simulink model "third"  (Simulink 8.6)
settings: Solver=ode23tb  StartTime=0.0  StopTime=3  MaxStep=1e-5  RelTol=1e-3
libraries: powerlib x6, simulink x2, powerlib_extras x1
settings Model: Creator=lenovo  LastModifiedBy=Administrator
settings OptimizationCC: InitFltsAndDblsToZero=on
settings DebuggingCC: SaveWithParameterizedLinksMsg=none  SignalResolutionControl=TryResolveAllWithWarning  MultiTaskDSMMsg=warning  MultiTaskCondExecSysMsg=none  FcnCallInpInsideContextMsg=UseLocalSettings
settings GRTTargetCC: TargetFcnLib=ansi_tfl_tmw.mat

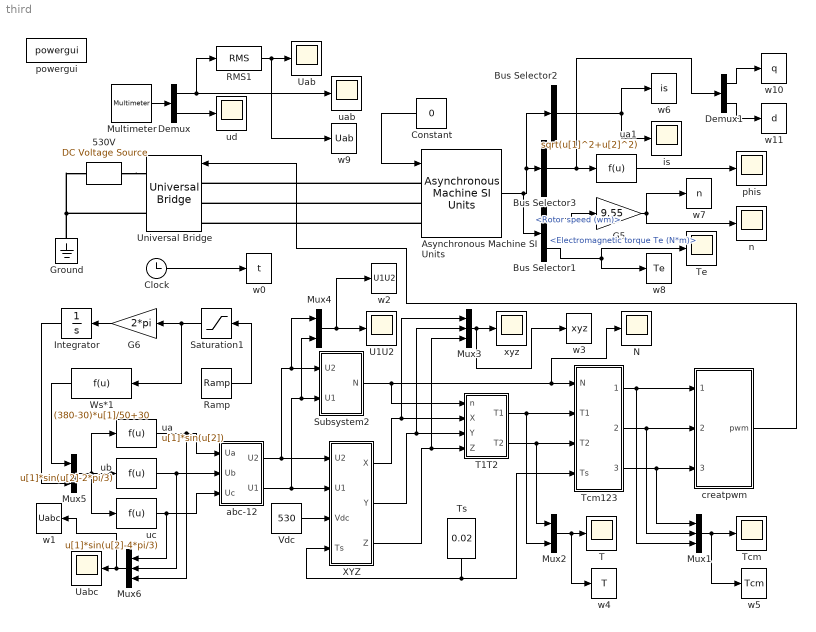
== system third ==
  530V : powerlib/Electrical Sources/DC Voltage Source  Amplitude=530  Measurements=Voltage
  Asynchronous Machine SI Units : powerlib/Machines/Asynchronous Machine SI Units  RotorType=Squirrel-cage  PresetModel=No  MechanicalLoad=Torque Tm  ShowDetailedParameters=on  ReferenceFrame=Rotor  Units=SI  MeasurementBus=off  NominalParameters=[2200 380 50]  Stator=[6.9 0.0455]  Rotor=[8.18 0.0455]  Cage1=[0.4155 0.002066]  Cage2=[0.4168 0.0003495]  Lm=1.0039  Mechanical=[0.02 0.005752 2]  PolePairs=2  InitialConditions="[ 1,0   0,0,0   0,0,0 ]"  SimulateSaturation=off  Saturation=[9.9249,19.6672,38.0377,51.3988,69.2824,105.1337,152.5532,214.2421,303.1917;230, 322, 414, 460, 506, 552, 598, 644, 690]  LoadFlowParameters=0  TsPowergui=0  TsBlock=-1  IterativeModel=Forward Euler  Pmec=1.492e+006
  Bus Selector1 : BusSelector  OutputSignals=Mechanical.Rotor speed (wm),Mechanical.Electromagnetic torque Te (N*m)
  Bus Selector2 : BusSelector  OutputSignals=Stator measurements.Stator current is_a (A),Stator measurements.Stator current is_b (A),Stator measurements.Stator current is_c (A)  OutputAsBus=on
  Bus Selector3 : BusSelector  OutputSignals=Stator measurements.Stator flux phis_q (V s),Stator measurements.Stator flux phis_d (V s)  OutputAsBus=on
  Clock : Clock
  Constant : Constant  Value=0
  Demux : Demux  Outputs=2
  Demux1 : Demux  Outputs=2
  G5 : Gain  Gain=9.55
  G6 : Gain  Gain=2*pi
  Ground : powerlib/Elements/Ground  LConnTagsString=a
  Integrator : Integrator
  Multimeter : powerlib/Measurements/Multimeter  PhasorSimulation=off  OutputType=Complex  sel=[7 11]  L=17  Gain=[1 1]  yselected={'Uab: Universal Bridge','Usrc: 530V'};  PSBOutputType=1  PSBequivalent=0  AxesSetting=[0,0.1,-100,100]  Display=0  SavedBlockNames=-11
  Mux1 : Mux  Inputs=3
  Mux2 : Mux  Inputs=2
  Mux3 : Mux  Inputs=3
  Mux4 : Mux  Inputs=2
  Mux5 : Mux  Inputs=2
  Mux6 : Mux  Inputs=3
  N : Scope
  RMS1 : powerlib_extras/Measurements/RMS  f1=60
  Ramp : simulink/Sources/Ramp  slope=50  start=0  X0=0
  Saturation1 : Saturate  UpperLimit=50
  Subsystem2 : Subsystem
  T : Scope
  T1T2 : Subsystem
  Tcm : Scope
  Tcm123 : Subsystem
  Te : Scope
  Ts : Constant  Value=0.02
  U1U2 : Scope
  Uab : Scope
  Uabc : Scope
  Universal Bridge : powerlib/Power Electronics/Universal Bridge  Arms=3  SnubberResistance=1e5  SnubberCapacitance=inf  Device=IGBT / Diodes  Ron=1e-3  Lon=0  ForwardVoltages="[  0  0  ]"  ForwardVoltage=0  GTOparameters=[ 10e-6 , 20e-6 ]  IGBTparameters=[ 1e-6 , 2e-6 ]  Measurements=All voltages and currents  Measurements_2=None  converterType=Rectifier
  Vdc : Constant  Value=530
  Ws*1 : Fcn  Expr=(380-30)*u[1]/50+30
  XYZ : Subsystem
  abc-12 : Subsystem
  creatpwm : Subsystem
  is : Scope
  n : Scope
  phis : Scope
  powergui : powerlib/powergui  SimulationMode=Continuous  SolverType=Tustin/Backward Euler (TBE)  SampleTime=1e-5  frequency=60  SPID=off  DisableSnubberDevices=off  DisableRonSwitches=off  DisableVfSwitches=off  SwTol=0  DisplayEquations=off  Interpol=off  ExternalGateDelay=off  methode=off  Ts=0  FunctionMessages=off  echomessages=off  HookPort=off  EnableUseOfTLC=off  x0status=blocks  frequencyindice=50  Pbase=100e6  ErrMax=1e-4  Iterations=50  UnitsV=kV  UnitsW=MW  buscounter=0  RestoreLinks=warning  ResistiveCurrentMeasurement=off  Frange=[0:2:500]  Ylog=off  Xlog=on  ShowGrid=off  save=off  variable=ZData  ZoomFFT=on  StartTime=0.0  cycles=1  DisplayStyle=1  fundamental=60  FreqAxis=off  MaxFrequency=1000  frequencyindicesteady=1  RmsSteady=1  display=off
  ua : Fcn  Expr=u[1]*sin(u[2])
  ua1 : Fcn  Expr=sqrt(u[1]^2+u[2]^2)
  uab : Scope
  ub : Fcn  Expr=u[1]*sin(u[2]-2*pi/3)
  uc : Fcn  Expr=u[1]*sin(u[2]-4*pi/3)
  ud : Scope
  w0 : ToWorkspace  VariableName=t  SampleTime=-1
  w1 : ToWorkspace  VariableName=Uabc  SampleTime=-1
  w10 : ToWorkspace  VariableName=q  SampleTime=-1
  w11 : ToWorkspace  VariableName=d  SampleTime=-1
  w2 : ToWorkspace  VariableName=U1U2  SampleTime=-1
  w3 : ToWorkspace  VariableName=xyz  SampleTime=-1
  w4 : ToWorkspace  VariableName=T  SampleTime=-1
  w5 : ToWorkspace  VariableName=Tcm  SampleTime=-1
  w6 : ToWorkspace  VariableName=is  SampleTime=-1
  w7 : ToWorkspace  VariableName=n  SampleTime=-1
  w8 : ToWorkspace  VariableName=Te  SampleTime=-1
  w9 : ToWorkspace  VariableName=Uab  SampleTime=-1
  xyz : Scope
  wires:
  Multimeter/1 -> Demux/1
  Demux/1 -> RMS1/1, uab/1
  Demux/2 -> ud/1
  Bus Selector2/1 -> is/1, w6/1
  Bus Selector1/1 -> G5/1  "<Rotor speed (wm)>"
  G5/1 -> w7/1, n/1
  Bus Selector1/2 -> Te/1, w8/1  "<Electromagnetic torque Te (N*m)>"
  Constant/1 -> Asynchronous Machine SI Units/1
  Ramp/1 -> Saturation1/1
  G6/1 -> Integrator/1
  Ws*1/1 -> Mux5/1
  Integrator/1 -> Mux5/2
  Mux5/1 -> ub/1, ua/1, uc/1
  Ts/1 -> XYZ/4(Ts), Tcm123/4(Ts)
  Vdc/1 -> XYZ/3(Vdc)
  Subsystem2/1(N) -> T1T2/1(n), Tcm123/1(N), N/1
  XYZ/1(X) -> T1T2/2(X), Mux3/1
  XYZ/2(Y) -> T1T2/3(Y), Mux3/2
  XYZ/3(Z) -> T1T2/4(Z), Mux3/3
  T1T2/1(T1) -> Tcm123/2(T1), Mux2/2
  T1T2/2(T2) -> Tcm123/3(T2), Mux2/1
  Tcm123/1(Tcm1) -> creatpwm/1(Tcm1), Mux1/3
  Tcm123/2(Tcm2) -> creatpwm/2(Tcm2), Mux1/2
  Tcm123/3(Tcm3) -> creatpwm/3(Tcm3), Mux1/1
  ua/1 -> abc-12/1(Ua), Mux6/3
  ub/1 -> abc-12/2(Ub), Mux6/2
  uc/1 -> abc-12/3(Uc), Mux6/1
  RMS1/1 -> Uab/1, w9/1
  abc-12/1(U2) -> XYZ/1(U2), Subsystem2/1(U2), Mux4/1
  abc-12/2(U1) -> XYZ/2(U1), Subsystem2/2(U1), Mux4/2
  Saturation1/1 -> G6/1, Ws*1/1
  Mux1/1 -> Tcm/1, w5/1
  Mux2/1 -> T/1, w4/1
  Mux3/1 -> w3/1, xyz/1
  Mux4/1 -> U1U2/1, w2/1
  Mux6/1 -> Uabc/1, w1/1
  Clock/1 -> w0/1
  ua1/1 -> phis/1
  creatpwm/1(pwm) -> Universal Bridge/1
  Bus Selector3/1 -> ua1/1, Demux1/1
  Demux1/1 -> w10/1
  Demux1/2 -> w11/1
  Asynchronous Machine SI Units/1 -> Bus Selector1/1, Bus Selector3/1, Bus Selector2/1
  connections:
  Asynchronous Machine SI Units/LConn1 -- Universal Bridge/LConn1
  Asynchronous Machine SI Units/LConn2 -- Universal Bridge/LConn2
  Asynchronous Machine SI Units/LConn3 -- Universal Bridge/LConn3
  Ground/LConn1 -- 530V/LConn1 -- Universal Bridge/RConn2
  530V/RConn1 -- Universal Bridge/RConn1

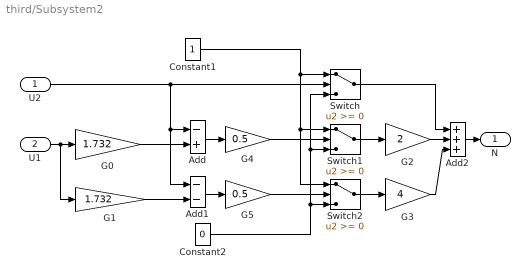
== system third/Subsystem2 ==
  U2 : Inport
  U1 : Inport  Port=2
  Add : Sum  Inputs=-+
  Add1 : Sum  Inputs=--
  Add2 : Sum  Inputs=+++
  Constant1 : Constant
  Constant2 : Constant  Value=0
  G0 : Gain  Gain=1.732
  G1 : Gain  Gain=1.732
  G2 : Gain  Gain=2
  G3 : Gain  Gain=4
  G4 : Gain  Gain=0.5
  G5 : Gain  Gain=0.5
  Switch : Switch
  Switch1 : Switch
  Switch2 : Switch
  N : Outport
  wires:
  Add2/1 -> N/1
  Switch/1 -> Add2/1
  G3/1 -> Add2/3
  G2/1 -> Add2/2
  Switch1/1 -> G2/1
  Switch2/1 -> G3/1
  Add1/1 -> G5/1
  Constant2/1 -> Switch2/3, Switch1/3, Switch/3
  Add/1 -> G4/1
  Constant1/1 -> Switch2/1, Switch1/1, Switch/1
  U2/1 -> Add1/1, Add/1, Switch/2
  G1/1 -> Add1/2
  U1/1 -> G1/1, G0/1
  G0/1 -> Add/2
  G4/1 -> Switch1/2
  G5/1 -> Switch2/2

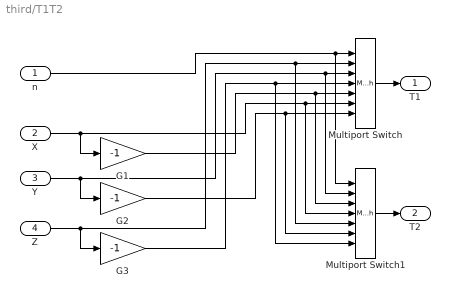
== system third/T1T2 ==
  n : Inport
  X : Inport  Port=2
  Y : Inport  Port=3
  Z : Inport  Port=4
  G1 : Gain  Gain=-1
  G2 : Gain  Gain=-1
  G3 : Gain  Gain=-1
  Multiport Switch : MultiPortSwitch  Inputs=6
  Multiport Switch1 : MultiPortSwitch  Inputs=6
  T1 : Outport
  T2 : Outport  Port=2
  wires:
  G2/1 -> Multiport Switch1/6, Multiport Switch/7
  G3/1 -> Multiport Switch1/7, Multiport Switch/4
  G1/1 -> Multiport Switch1/3, Multiport Switch/5
  Z/1 -> Multiport Switch1/5, Multiport Switch/2, G3/1
  Y/1 -> Multiport Switch1/2, Multiport Switch/3, G2/1
  X/1 -> Multiport Switch1/4, Multiport Switch/6, G1/1
  n/1 -> Multiport Switch1/1, Multiport Switch/1
  Multiport Switch1/1 -> T2/1
  Multiport Switch/1 -> T1/1

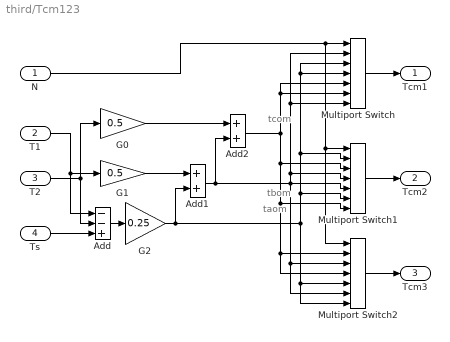
== system third/Tcm123 ==
  note: taom
  note: tbom
  note: tcom
  N : Inport
  T1 : Inport  Port=2
  T2 : Inport  Port=3
  Ts : Inport  Port=4
  Add : Sum  Inputs=--+
  Add1 : Sum
  Add2 : Sum
  G0 : Gain  Gain=0.5
  G1 : Gain  Gain=0.5
  G2 : Gain  Gain=0.25
  Multiport Switch : MultiPortSwitch  Inputs=6
  Multiport Switch1 : MultiPortSwitch  Inputs=6
  Multiport Switch2 : MultiPortSwitch  Inputs=6
  Tcm1 : Outport
  Tcm2 : Outport  Port=2
  Tcm3 : Outport  Port=3
  wires:
  Add2/1 -> Multiport Switch1/3, Multiport Switch2/4, Multiport Switch2/2, Multiport Switch1/7, Multiport Switch/5, Multiport Switch/6
  Add1/1 -> Multiport Switch2/6, Multiport Switch2/3, Multiport Switch1/5, Multiport Switch1/4, Multiport Switch/2, Multiport Switch/7, Add2/2
  G2/1 -> Multiport Switch2/5, Multiport Switch2/7, Multiport Switch1/6, Multiport Switch1/2, Multiport Switch/4, Multiport Switch/3, Add1/2
  G1/1 -> Add1/1
  G0/1 -> Add2/1
  Add/1 -> G2/1
  Ts/1 -> Add/3
  T2/1 -> Add/2, G0/1
  T1/1 -> Add/1, G1/1
  Multiport Switch2/1 -> Tcm3/1
  Multiport Switch1/1 -> Tcm2/1
  N/1 -> Multiport Switch/1, Multiport Switch2/1, Multiport Switch1/1
  Multiport Switch/1 -> Tcm1/1

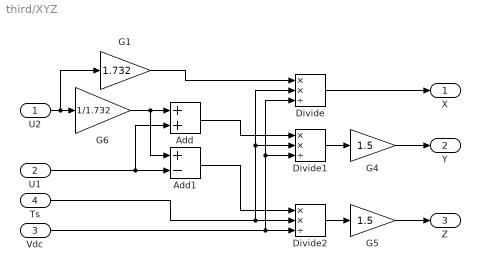
== system third/XYZ ==
  U2 : Inport
  U1 : Inport  Port=2
  Vdc : Inport  Port=3
  Ts : Inport  Port=4
  Add : Sum
  Add1 : Sum  Inputs=+-
  Divide : Product  Inputs=**/
  Divide1 : Product  Inputs=**/
  Divide2 : Product  Inputs=**/
  G1 : Gain  Gain=1.732
  G4 : Gain  Gain=1.5
  G5 : Gain  Gain=1.5
  G6 : Gain  Gain=1/1.732
  X : Outport
  Y : Outport  Port=2
  Z : Outport  Port=3
  wires:
  Divide/1 -> X/1
  G4/1 -> Y/1
  G5/1 -> Z/1
  Divide2/1 -> G5/1
  Divide1/1 -> G4/1
  Vdc/1 -> Divide/3, Divide1/3, Divide2/3
  Ts/1 -> Divide/2, Divide1/2, Divide2/2
  Add1/1 -> Divide2/1
  Add/1 -> Divide1/1
  G1/1 -> Divide/1
  U1/1 -> Add1/2, Add/2
  U2/1 -> G1/1, G6/1
  G6/1 -> Add/1, Add1/1

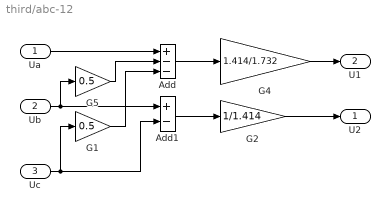
== system third/abc-12 ==
  Ua : Inport
  Ub : Inport  Port=2
  Uc : Inport  Port=3
  Add : Sum  Inputs=+--
  Add1 : Sum  Inputs=+-
  G1 : Gain  Gain=0.5
  G2 : Gain  Gain=1/1.414
  G4 : Gain  Gain=1.414/1.732
  G5 : Gain  Gain=0.5
  U2 : Outport
  U1 : Outport  Port=2
  wires:
  Ua/1 -> Add/1
  Ub/1 -> G5/1, Add1/1
  G2/1 -> U2/1
  Uc/1 -> G1/1, Add1/2
  Add/1 -> G4/1
  G4/1 -> U1/1
  Add1/1 -> G2/1
  G5/1 -> Add/2
  G1/1 -> Add/3

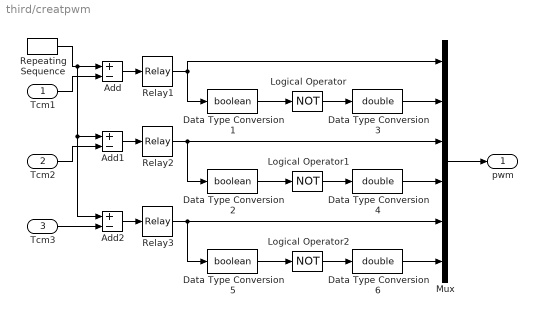
== system third/creatpwm ==
  Tcm1 : Inport
  Tcm2 : Inport  Port=2
  Tcm3 : Inport  Port=3
  Add : Sum  Inputs=+-
  Add1 : Sum  Inputs=+-
  Add2 : Sum  Inputs=+-
  Data Type Conversion1 : DataTypeConversion  OutDataTypeStr=boolean
  Data Type Conversion2 : DataTypeConversion  OutDataTypeStr=boolean
  Data Type Conversion3 : DataTypeConversion  OutDataTypeStr=double
  Data Type Conversion4 : DataTypeConversion  OutDataTypeStr=double
  Data Type Conversion5 : DataTypeConversion  OutDataTypeStr=boolean
  Data Type Conversion6 : DataTypeConversion  OutDataTypeStr=double
  Logical Operator : Logic  Operator=NOT  AllPortsSameDT=off  OutDataTypeStr=boolean
  Logical Operator1 : Logic  Operator=NOT  AllPortsSameDT=off  OutDataTypeStr=boolean
  Logical Operator2 : Logic  Operator=NOT  AllPortsSameDT=off  OutDataTypeStr=boolean
  Mux : Mux  Inputs=6
  Relay1 : Relay
  Relay2 : Relay
  Relay3 : Relay
  Repeating Sequence : simulink/Sources/Repeating Sequence  rep_seq_t=[0 5e-4]  rep_seq_y=[-0.003 0.013]
  pwm : Outport
  wires:
  Mux/1 -> pwm/1
  Tcm1/1 -> Add/2
  Logical Operator2/1 -> Data Type Conversion6/1
  Data Type Conversion5/1 -> Logical Operator2/1
  Logical Operator1/1 -> Data Type Conversion4/1
  Data Type Conversion2/1 -> Logical Operator1/1
  Logical Operator/1 -> Data Type Conversion3/1
  Data Type Conversion1/1 -> Logical Operator/1
  Relay1/1 -> Mux/1, Data Type Conversion1/1
  Relay3/1 -> Mux/5, Data Type Conversion5/1
  Relay2/1 -> Mux/3, Data Type Conversion2/1
  Add2/1 -> Relay3/1
  Add1/1 -> Relay2/1
  Add/1 -> Relay1/1
  Tcm3/1 -> Add2/2
  Tcm2/1 -> Add1/2
  Data Type Conversion3/1 -> Mux/2
  Data Type Conversion4/1 -> Mux/4
  Data Type Conversion6/1 -> Mux/6
  Repeating Sequence/1 -> Add/1, Add1/1, Add2/1
